simulink model "LogicalArch"  (R2025a)
settings: Solver=FixedStepDiscrete  StartTime=0.0  StopTime=10.0  RelTol=1e-3
undefined symbols (not defined in the file): D1, P
settings Model: DataDictionary=MotionController.sldd  Creator=mfussi  LastModifiedBy=mfussi
settings OptimizationCC: DefaultParameterBehavior=Inlined  EnhancedBackFolding=on  PassReuseOutputArgsAs=Individual arguments  ZeroExternalMemoryAtStartup=off  ZeroInternalMemoryAtStartup=off  OptimizeBlockOrder=speed  DifferentSizesBufferReuse=on  OptimizationCustomize=off  EfficientTunableParamExpr=on
settings DebuggingCC: ParameterTunabilityLossMsg=error
settings SFSimCC: MATLABDynamicMemAlloc=off
settings RTWCC: SystemTargetFile=ert.tlc  TemplateMakefile=ert_default_tmf  Description=Embedded Coder
settings CodeAppCC: ForceParamTrailComments=on  IgnoreCustomStorageClasses=off  OperatorAnnotations=on  SimulinkDataObjDesc=on  SFDataObjDesc=on  InsertBlockDesc=on
settings ERTTargetCC: ExtModeTransport=0.0  ExtModeStaticAlloc=off  ExtModeMexFile=ext_comm  ExtModeIntrfLevel=Level1  ERTCustomFileTemplate=example_file_process.tlc  TargetLangStandard=C99 (ISO)  GenerateSampleERTMain=on

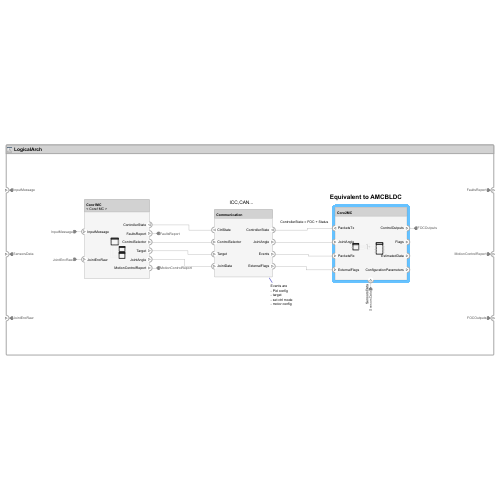
[thumbnail: Simulink's stored preview of the top-level diagram]
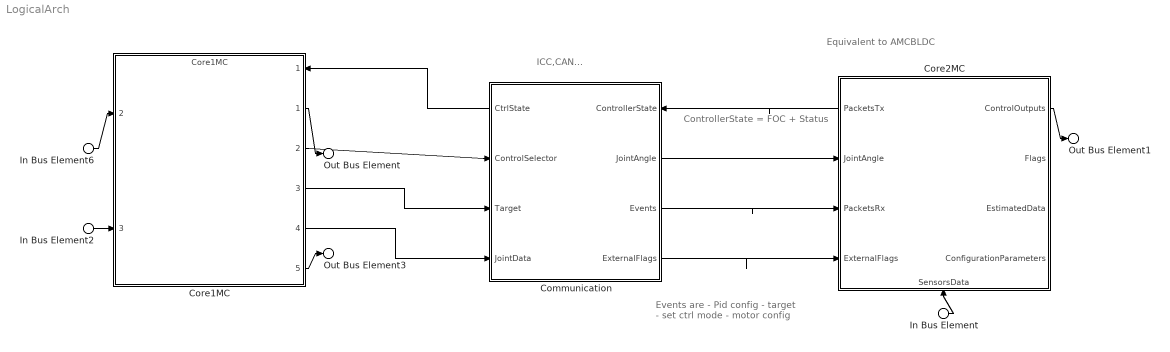
== system LogicalArch ==
  note: ControllerState = FOC + Status
  note: Events are
      | - Pid config
      | - target
      | - set ctrl mode
      | - motor config
  note: ICC,CAN...
  note: Equivalent to AMCBLDC
  In Bus Element6 : Inport  PortName=InputMessage
  In Bus Element : Inport  Port=2  PortName=SensorsData
  In Bus Element2 : Inport  Port=3  PortName=JointEncRaw
  Communication : Subsystem
      settings: PortSchema="{\"entries\":[{\"content\":{\"headerSize\":26,\"margin\":15,\"minimumSpacing\":25,\"sides\":[{\"content\":{\"connectorIds\":[\"Out1\",\"In2\",\"In3\",\"In4\"]},\"type\":\"ConnectorPlacement.EquallySpacedRectSide\",\"uuid\":\"fe08bce5-e822-4f40-96c8-d2e734a990df\"},{\"content\":{\"connectorIds\":[\"In1\",\"Out2\",\"Out4\",\"Out3\"],\"side\":\"RIGHT\"},\"type\":\"ConnectorPlacement.EquallySpacedRectSide\",\"uuid\":\"919d1c7d-1061-4f77-a351-e4b0010947a9\"},{\"content\":{\"side\":\"TOP\"},\"type\":\"ConnectorPlacement.EquallySpacedRectSide\",\"uuid\":\"ced767b1-6519-463a-89bd-856cb58a8166\"}]},\"type\":\"ConnectorPlacement.EquallySpacedConnector\",\"uuid\":\"cdf15350-aaf1-41b4-b116-0e65771ee3f3\"}],\"packageUris\":[\"http://schema.mathworks.com/mf0/Connector/R2020b\"],\"version\":\"1.0\"}"
  Core1MC : ModelReference  ModelNameDialog=Core1MC.slx  SimulationMode=Normal  ScheduleRates=on  ModelReferenceVersion=1.2
      settings: PortSchema="{\"entries\":[{\"content\":{\"headerSize\":38,\"margin\":15,\"minimumSpacing\":25,\"sides\":[{\"content\":{\"connectorIds\":[\"In2\",\"In3\"]},\"type\":\"ConnectorPlacement.EquallySpacedRectSide\",\"uuid\":\"f116faee-1f2a-4df9-9539-2b4210afeefe\"},{\"content\":{\"connectorIds\":[\"In1\",\"Out1\",\"Out2\",\"Out3\",\"Out4\",\"Out5\"],\"side\":\"RIGHT\"},\"type\":\"ConnectorPlacement.EquallySpacedRectSide\",\"uuid\":\"15bee73e-70ab-48d7-8ec7-8f9a927bc16b\"},{\"content\":{\"side\":\"TOP\"},\"type\":\"ConnectorPlacement.EquallySpacedRectSide\",\"uuid\":\"028c131f-52af-49f4-b789-e2e615b5b11c\"}]},\"type\":\"ConnectorPlacement.EquallySpacedConnector\",\"uuid\":\"2ab3b17c-88dc-4a6c-bd49-4ef3d2b344d3\"}],\"packageUris\":[\"http://schema.mathworks.com/mf0/Connector/R2020b\"],\"version\":\"1.0\"}"
  Core2MC : Subsystem
      settings: PortSchema="{\"entries\":[{\"content\":{\"headerSize\":26,\"margin\":15,\"minimumSpacing\":25,\"sides\":[{\"content\":{\"connectorIds\":[\"Out1\",\"In1\",\"In3\",\"In2\"]},\"type\":\"ConnectorPlacement.EquallySpacedRectSide\",\"uuid\":\"8a080317-9bcc-45dd-ad9c-7d7a1d267dc1\"},{\"content\":{\"connectorIds\":[\"Out2\",\"Out3\",\"Out4\",\"Out5\"],\"side\":\"RIGHT\"},\"type\":\"ConnectorPlacement.EquallySpacedRectSide\",\"uuid\":\"40b95da5-0e38-4058-8ebd-913319e6fe12\"},{\"content\":{\"side\":\"TOP\"},\"type\":\"ConnectorPlacement.EquallySpacedRectSide\",\"uuid\":\"880187c3-7d3f-4130-85c8-9403ff1f590f\"},{\"content\":{\"connectorIds\":[\"In4\"],\"side\":\"BOTTOM\"},\"type\":\"ConnectorPlacement.EquallySpacedRectSide\",\"uuid\":\"cb8d9f13-ba0e-48de-be5c-602b33a49657\"}]},\"type\":\"ConnectorPlacement.EquallySpacedConnector\",\"uuid\":\"156347fc-2d8f-4aa4-81e2-6bd9fedc9a5a\"}],\"packageUris\":[\"http://schema.mathworks.com/mf0/Connector/R2020b\"],\"version\":\"1.0\"}"
  Out Bus Element : Outport  PortName=FaultsReport
  Out Bus Element3 : Outport  Port=2  PortName=MotionControlReport
  Out Bus Element1 : Outport  Port=3  PortName=FOCOutputs
  wires:
  Communication/2(JointAngle) -> Core2MC/1(JointAngle)
  Communication/4(Events) -> Core2MC/3(PacketsRx)
  Core2MC/1(PacketsTx) -> Communication/1(ControllerState)
  Core1MC/2 -> Communication/2(ControlSelector)
  Core1MC/3 -> Communication/3(Target)
  Core1MC/4 -> Communication/4(JointData)
  Communication/1(CtrlState) -> Core1MC/1
  In Bus Element6/1 -> Core1MC/2
  In Bus Element2/1 -> Core1MC/3
  In Bus Element/1 -> Core2MC/4(SensorsData)
  Communication/3(ExternalFlags) -> Core2MC/2(ExternalFlags)
  Core2MC/2(ControlOutputs) -> Out Bus Element1/1
  Core1MC/1 -> Out Bus Element/1
  Core1MC/5 -> Out Bus Element3/1

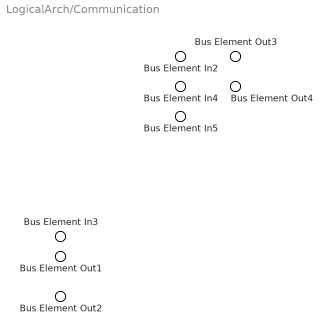
== system LogicalArch/Communication ==
  Bus Element In5 : Inport  PortName=ControllerState
  Bus Element In2 : Inport  Port=2  PortName=ControlSelector
  Bus Element In4 : Inport  Port=3  PortName=Target
  Bus Element In3 : Inport  Port=4  PortName=JointData
  Bus Element Out3 : Outport  PortName=CtrlState
  Bus Element Out1 : Outport  Port=2  PortName=JointAngle
  Bus Element Out4 : Outport  Port=3  PortName=ExternalFlags
  Bus Element Out2 : Outport  Port=4  PortName=Events

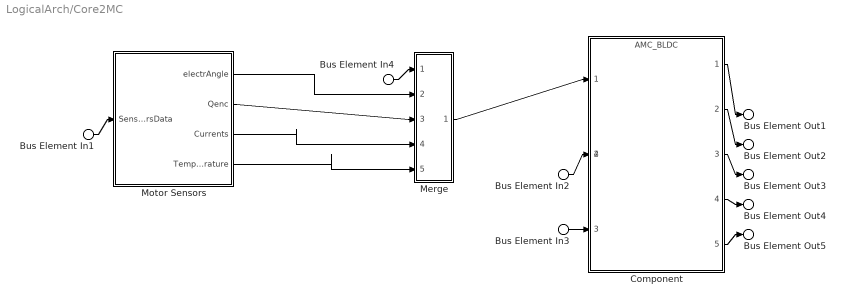
== system LogicalArch/Core2MC ==
  Bus Element In4 : Inport  PortName=JointAngle
  Bus Element In2 : Inport  Port=2  PortName=ExternalFlags
  Bus Element In3 : Inport  Port=3  PortName=PacketsRx
  Bus Element In1 : Inport  Port=4  PortName=SensorsData
  Component : ModelReference  ModelNameDialog=AMC_BLDC.slx  SimulationMode=Normal  ScheduleRates=on  ModelEventPortInfo=P:D1[-2][0][0]  ModelReferenceVersion=10.21
      settings: PortSchema="{\"entries\":[{\"content\":{\"headerSize\":38,\"margin\":15,\"minimumSpacing\":25,\"sides\":[{\"content\":{\"connectorIds\":[\"In1\",\"In2\",\"In3\"]},\"type\":\"ConnectorPlacement.EquallySpacedRectSide\",\"uuid\":\"f116faee-1f2a-4df9-9539-2b4210afeefe\"},{\"content\":{\"connectorIds\":[\"Out1\",\"Out2\",\"Out3\",\"Out4\",\"Out5\"],\"side\":\"RIGHT\"},\"type\":\"ConnectorPlacement.EquallySpacedRectSide\",\"uuid\":\"15bee73e-70ab-48d7-8ec7-8f9a927bc16b\"},{\"content\":{\"side\":\"TOP\"},\"type\":\"ConnectorPlacement.EquallySpacedRectSide\",\"uuid\":\"028c131f-52af-49f4-b789-e2e615b5b11c\"},{\"content\":{\"connectorIds\":[\"In4\"],\"side\":\"HIDDEN\"},\"type\":\"ConnectorPlacement.EquallySpacedRectSide\",\"uuid\":\"a9e6405e-7b1c-4ea5-9964-f820342ca78f\"}]},\"type\":\"ConnectorPlacement.EquallySpacedConnector\",\"uuid\":\"2ab3b17c-88dc-4a6c-bd49-4ef3d2b344d3\"}],\"packageUris\":[\"http://schema.mathworks.com/mf0/Connector/R2020b\"],\"version\":\"1.0\"}"
  Merge : Subsystem
      settings: PortSchema="{\"entries\":[{\"content\":{\"margin\":10,\"minimumSpacing\":15,\"sides\":[{\"content\":{\"connectorIds\":[\"In1\",\"In2\",\"In3\",\"In4\",\"In5\"]},\"type\":\"ConnectorPlacement.EquallySpacedRectSide\",\"uuid\":\"b721ea92-b23b-49c6-b256-e109cfde6d9a\"},{\"content\":{\"connectorIds\":[\"Out1\"],\"side\":\"RIGHT\"},\"type\":\"ConnectorPlacement.EquallySpacedRectSide\",\"uuid\":\"01ecff02-faf6-44fc-85cd-eb338f239b8b\"},{\"content\":{\"side\":\"TOP\"},\"type\":\"ConnectorPlacement.EquallySpacedRectSide\",\"uuid\":\"b7f583c7-535b-43ea-9e2b-1d6295f5e2cc\"}]},\"type\":\"ConnectorPlacement.EquallySpacedConnector\",\"uuid\":\"374a74ae-7551-4f3a-8e98-a33b88a70ffb\"}],\"packageUris\":[\"http://schema.mathworks.com/mf0/Connector/R2020b\"],\"version\":\"1.0\"}"
  Motor Sensors : Subsystem
      settings: PortSchema="{\"entries\":[{\"content\":{\"headerSize\":26,\"margin\":15,\"minimumSpacing\":25,\"sides\":[{\"content\":{\"connectorIds\":[\"In1\"]},\"type\":\"ConnectorPlacement.EquallySpacedRectSide\",\"uuid\":\"342e77a0-fe02-4293-9b8f-d7b4d9d1e449\"},{\"content\":{\"connectorIds\":[\"Out2\",\"Out3\",\"Out4\",\"Out1\"],\"side\":\"RIGHT\"},\"type\":\"ConnectorPlacement.EquallySpacedRectSide\",\"uuid\":\"44d1e335-dcc4-49cc-8b5e-810d6adc679c\"},{\"content\":{\"side\":\"TOP\"},\"type\":\"ConnectorPlacement.EquallySpacedRectSide\",\"uuid\":\"025af28e-bbdd-4ddf-9ce9-395878e2a87b\"},{\"content\":{\"side\":\"BOTTOM\"},\"type\":\"ConnectorPlacement.EquallySpacedRectSide\",\"uuid\":\"55873401-33e6-4ccb-9330-bdb43b58e7a9\"}]},\"type\":\"ConnectorPlacement.EquallySpacedConnector\",\"uuid\":\"48047874-33f0-4080-8e53-46ed85469308\"}],\"packageUris\":[\"http://schema.mathworks.com/mf0/Connector/R2020b\"],\"version\":\"1.0\"}"
  Bus Element Out5 : Outport  PortName=PacketsTx
  Bus Element Out1 : Outport  Port=2  PortName=ControlOutputs
  Bus Element Out3 : Outport  Port=3  PortName=Flags
  Bus Element Out4 : Outport  Port=4  PortName=EstimatedData
  Bus Element Out2 : Outport  Port=5  PortName=ConfigurationParameters
  wires:
  Bus Element In1/1 -> Motor Sensors/1(SensorsData)
  Motor Sensors/2(electrAngle) -> Merge/2(electrAngle)
  Motor Sensors/4(Currents) -> Merge/4(Currents)
  Motor Sensors/3(Qenc) -> Merge/3(Qenc)
  Motor Sensors/1(Temperature) -> Merge/5(Temperature)
  Merge/1(ProcessedSensors) -> Component/1
  Bus Element In2/1 -> Component/2
  Component/1 -> Bus Element Out1/1
  Component/2 -> Bus Element Out2/1
  Component/3 -> Bus Element Out3/1
  Component/4 -> Bus Element Out4/1
  Component/5 -> Bus Element Out5/1
  Bus Element In3/1 -> Component/3
  Bus Element In4/1 -> Merge/1(JointAngle)

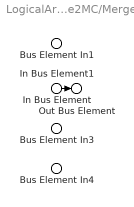
== system LogicalArch/Core2MC/Merge ==
  Bus Element In1 : Inport  PortName=JointAngle
  In Bus Element : Inport  Port=2  PortName=electrAngle
  In Bus Element1 : Inport  Port=3  PortName=Qenc
  Bus Element In3 : Inport  Port=4  PortName=Currents
  Bus Element In4 : Inport  Port=5  PortName=Temperature
  Out Bus Element : Outport  PortName=ProcessedSensors
  wires:
  In Bus Element/1 -> Out Bus Element/1

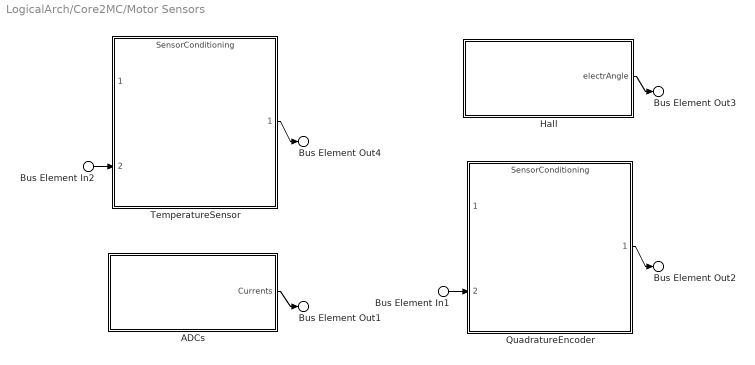
== system LogicalArch/Core2MC/Motor Sensors ==
  Bus Element In1 : Inport  PortName=SensorsData
  Bus Element In2 : Inport  PortName=SensorsData
  ADCs : Subsystem
      settings: PortSchema="{\"entries\":[{\"content\":{\"headerSize\":26,\"margin\":15,\"minimumSpacing\":25,\"sides\":[{\"content\":{},\"type\":\"ConnectorPlacement.EquallySpacedRectSide\",\"uuid\":\"15e2ce74-797f-4db5-be27-721c76b78586\"},{\"content\":{\"connectorIds\":[\"Out1\"],\"side\":\"RIGHT\"},\"type\":\"ConnectorPlacement.EquallySpacedRectSide\",\"uuid\":\"77d311f1-c2d5-4f29-9693-3cfe7ff3c66f\"},{\"content\":{\"side\":\"TOP\"},\"type\":\"ConnectorPlacement.EquallySpacedRectSide\",\"uuid\":\"0ad7fd31-5953-422f-9352-5b06c9bff885\"}]},\"type\":\"ConnectorPlacement.EquallySpacedConnector\",\"uuid\":\"9e5c4c0a-c38e-4cf1-bd50-bfe5cf75fba8\"}],\"packageUris\":[\"http://schema.mathworks.com/mf0/Connector/R2020b\"],\"version\":\"1.0\"}"
  Hall : Subsystem
      settings: PortSchema="{\"entries\":[{\"content\":{\"headerSize\":26,\"margin\":15,\"minimumSpacing\":25,\"sides\":[{\"content\":{},\"type\":\"ConnectorPlacement.EquallySpacedRectSide\",\"uuid\":\"fe08bce5-e822-4f40-96c8-d2e734a990df\"},{\"content\":{\"connectorIds\":[\"Out1\"],\"side\":\"RIGHT\"},\"type\":\"ConnectorPlacement.EquallySpacedRectSide\",\"uuid\":\"919d1c7d-1061-4f77-a351-e4b0010947a9\"},{\"content\":{\"side\":\"TOP\"},\"type\":\"ConnectorPlacement.EquallySpacedRectSide\",\"uuid\":\"ced767b1-6519-463a-89bd-856cb58a8166\"}]},\"type\":\"ConnectorPlacement.EquallySpacedConnector\",\"uuid\":\"cdf15350-aaf1-41b4-b116-0e65771ee3f3\"}],\"packageUris\":[\"http://schema.mathworks.com/mf0/Connector/R2020b\"],\"version\":\"1.0\"}"
  QuadratureEncoder : ModelReference  ModelNameDialog=SensorConditioning.slx  SimulationMode=Normal  ScheduleRates=on  ModelReferenceVersion=1.2
      settings: PortSchema="{\"entries\":[{\"content\":{\"headerSize\":38,\"margin\":15,\"minimumSpacing\":25,\"sides\":[{\"content\":{\"connectorIds\":[\"In1\",\"In2\"]},\"type\":\"ConnectorPlacement.EquallySpacedRectSide\",\"uuid\":\"6d6857fa-f5c9-43b4-a306-0920391a2fd0\"},{\"content\":{\"connectorIds\":[\"Out1\"],\"side\":\"RIGHT\"},\"type\":\"ConnectorPlacement.EquallySpacedRectSide\",\"uuid\":\"4567897e-6982-4f2c-af43-5ed4bc8792a2\"},{\"content\":{\"side\":\"TOP\"},\"type\":\"ConnectorPlacement.EquallySpacedRectSide\",\"uuid\":\"b9101744-fe35-433d-bb4c-e7449aefab81\"}]},\"type\":\"ConnectorPlacement.EquallySpacedConnector\",\"uuid\":\"96c92cf5-557b-4ff0-b6b4-f2ae6063b6b3\"}],\"packageUris\":[\"http://schema.mathworks.com/mf0/Connector/R2020b\"],\"version\":\"1.0\"}"
  TemperatureSensor : ModelReference  ModelNameDialog=SensorConditioning.slx  SimulationMode=Normal  ScheduleRates=on  ModelReferenceVersion=1.2
      settings: PortSchema="{\"entries\":[{\"content\":{\"headerSize\":38,\"margin\":15,\"minimumSpacing\":25,\"sides\":[{\"content\":{\"connectorIds\":[\"In1\",\"In2\"]},\"type\":\"ConnectorPlacement.EquallySpacedRectSide\",\"uuid\":\"6d6857fa-f5c9-43b4-a306-0920391a2fd0\"},{\"content\":{\"connectorIds\":[\"Out1\"],\"side\":\"RIGHT\"},\"type\":\"ConnectorPlacement.EquallySpacedRectSide\",\"uuid\":\"4567897e-6982-4f2c-af43-5ed4bc8792a2\"},{\"content\":{\"side\":\"TOP\"},\"type\":\"ConnectorPlacement.EquallySpacedRectSide\",\"uuid\":\"b9101744-fe35-433d-bb4c-e7449aefab81\"}]},\"type\":\"ConnectorPlacement.EquallySpacedConnector\",\"uuid\":\"96c92cf5-557b-4ff0-b6b4-f2ae6063b6b3\"}],\"packageUris\":[\"http://schema.mathworks.com/mf0/Connector/R2020b\"],\"version\":\"1.0\"}"
  Bus Element Out4 : Outport  PortName=Temperature
  Bus Element Out3 : Outport  Port=2  PortName=electrAngle
  Bus Element Out2 : Outport  Port=3  PortName=Qenc
  Bus Element Out1 : Outport  Port=4  PortName=Currents
  wires:
  ADCs/1(Currents) -> Bus Element Out1/1
  Hall/1(electrAngle) -> Bus Element Out3/1
  TemperatureSensor/1 -> Bus Element Out4/1
  QuadratureEncoder/1 -> Bus Element Out2/1
  Bus Element In1/1 -> QuadratureEncoder/2
  Bus Element In2/1 -> TemperatureSensor/2

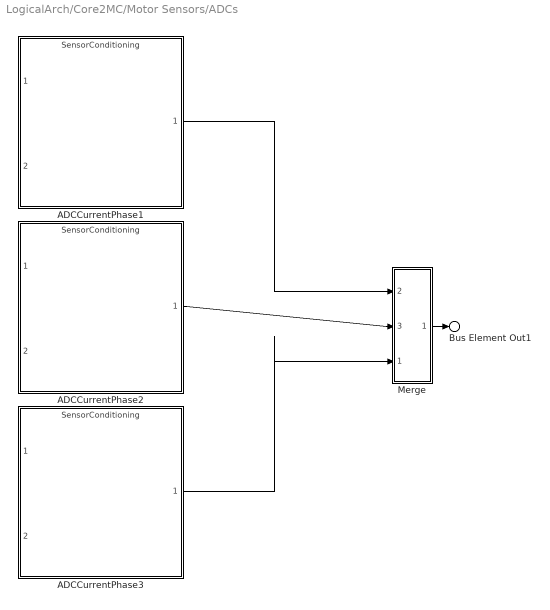
== system LogicalArch/Core2MC/Motor Sensors/ADCs ==
  ADCCurrentPhase1 : ModelReference  ModelNameDialog=SensorConditioning.slx  SimulationMode=Normal  ScheduleRates=on  ModelReferenceVersion=1.2
      settings: PortSchema="{\"entries\":[{\"content\":{\"headerSize\":38,\"margin\":15,\"minimumSpacing\":25,\"sides\":[{\"content\":{\"connectorIds\":[\"In1\",\"In2\"]},\"type\":\"ConnectorPlacement.EquallySpacedRectSide\",\"uuid\":\"6d6857fa-f5c9-43b4-a306-0920391a2fd0\"},{\"content\":{\"connectorIds\":[\"Out1\"],\"side\":\"RIGHT\"},\"type\":\"ConnectorPlacement.EquallySpacedRectSide\",\"uuid\":\"4567897e-6982-4f2c-af43-5ed4bc8792a2\"},{\"content\":{\"side\":\"TOP\"},\"type\":\"ConnectorPlacement.EquallySpacedRectSide\",\"uuid\":\"b9101744-fe35-433d-bb4c-e7449aefab81\"}]},\"type\":\"ConnectorPlacement.EquallySpacedConnector\",\"uuid\":\"96c92cf5-557b-4ff0-b6b4-f2ae6063b6b3\"}],\"packageUris\":[\"http://schema.mathworks.com/mf0/Connector/R2020b\"],\"version\":\"1.0\"}"
  ADCCurrentPhase2 : ModelReference  ModelNameDialog=SensorConditioning.slx  SimulationMode=Normal  ScheduleRates=on  ModelReferenceVersion=1.2
      settings: PortSchema="{\"entries\":[{\"content\":{\"headerSize\":38,\"margin\":15,\"minimumSpacing\":25,\"sides\":[{\"content\":{\"connectorIds\":[\"In1\",\"In2\"]},\"type\":\"ConnectorPlacement.EquallySpacedRectSide\",\"uuid\":\"6d6857fa-f5c9-43b4-a306-0920391a2fd0\"},{\"content\":{\"connectorIds\":[\"Out1\"],\"side\":\"RIGHT\"},\"type\":\"ConnectorPlacement.EquallySpacedRectSide\",\"uuid\":\"4567897e-6982-4f2c-af43-5ed4bc8792a2\"},{\"content\":{\"side\":\"TOP\"},\"type\":\"ConnectorPlacement.EquallySpacedRectSide\",\"uuid\":\"b9101744-fe35-433d-bb4c-e7449aefab81\"}]},\"type\":\"ConnectorPlacement.EquallySpacedConnector\",\"uuid\":\"96c92cf5-557b-4ff0-b6b4-f2ae6063b6b3\"}],\"packageUris\":[\"http://schema.mathworks.com/mf0/Connector/R2020b\"],\"version\":\"1.0\"}"
  ADCCurrentPhase3 : ModelReference  ModelNameDialog=SensorConditioning.slx  SimulationMode=Normal  ScheduleRates=on  ModelReferenceVersion=1.2
      settings: PortSchema="{\"entries\":[{\"content\":{\"headerSize\":38,\"margin\":15,\"minimumSpacing\":25,\"sides\":[{\"content\":{\"connectorIds\":[\"In1\",\"In2\"]},\"type\":\"ConnectorPlacement.EquallySpacedRectSide\",\"uuid\":\"6d6857fa-f5c9-43b4-a306-0920391a2fd0\"},{\"content\":{\"connectorIds\":[\"Out1\"],\"side\":\"RIGHT\"},\"type\":\"ConnectorPlacement.EquallySpacedRectSide\",\"uuid\":\"4567897e-6982-4f2c-af43-5ed4bc8792a2\"},{\"content\":{\"side\":\"TOP\"},\"type\":\"ConnectorPlacement.EquallySpacedRectSide\",\"uuid\":\"b9101744-fe35-433d-bb4c-e7449aefab81\"}]},\"type\":\"ConnectorPlacement.EquallySpacedConnector\",\"uuid\":\"96c92cf5-557b-4ff0-b6b4-f2ae6063b6b3\"}],\"packageUris\":[\"http://schema.mathworks.com/mf0/Connector/R2020b\"],\"version\":\"1.0\"}"
  Merge : Subsystem
      settings: PortSchema="{\"entries\":[{\"content\":{\"margin\":10,\"minimumSpacing\":15,\"sides\":[{\"content\":{\"connectorIds\":[\"In2\",\"In3\",\"In1\"]},\"type\":\"ConnectorPlacement.EquallySpacedRectSide\",\"uuid\":\"7f12f04c-5461-4836-a734-adc2bf884dca\"},{\"content\":{\"connectorIds\":[\"Out1\"],\"side\":\"RIGHT\"},\"type\":\"ConnectorPlacement.EquallySpacedRectSide\",\"uuid\":\"3e6e724d-a2e9-44fd-aa47-81a7ca7b1e30\"},{\"content\":{\"side\":\"TOP\"},\"type\":\"ConnectorPlacement.EquallySpacedRectSide\",\"uuid\":\"a6eebf31-70f0-4364-98fd-7bcbddea794c\"},{\"content\":{\"side\":\"BOTTOM\"},\"type\":\"ConnectorPlacement.EquallySpacedRectSide\",\"uuid\":\"70e5c21f-7bf5-4633-9f55-33f7ef1ae04e\"}]},\"type\":\"ConnectorPlacement.EquallySpacedConnector\",\"uuid\":\"958be322-7dc9-477a-a570-cb6c9a7ff655\"}],\"packageUris\":[\"http://schema.mathworks.com/mf0/Connector/R2020b\"],\"version\":\"1.0\"}"
  Bus Element Out1 : Outport  PortName=Currents
  wires:
  Merge/1(Currents) -> Bus Element Out1/1
  ADCCurrentPhase1/1 -> Merge/2("CurrentPhase1 ")
  ADCCurrentPhase2/1 -> Merge/3(CurrentPhase2)
  ADCCurrentPhase3/1 -> Merge/1(CurrentPhase3)

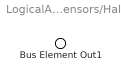
== system LogicalArch/Core2MC/Motor Sensors/Hall ==
  Bus Element Out1 : Outport  PortName=electrAngle

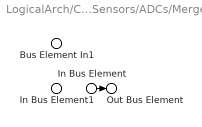
== system LogicalArch/Core2MC/Motor Sensors/ADCs/Merge ==
  Bus Element In1 : Inport  PortName=CurrentPhase3
  In Bus Element : Inport  Port=2  PortName=CurrentPhase1
  In Bus Element1 : Inport  Port=3  PortName=CurrentPhase2
  Out Bus Element : Outport  PortName=Currents
  wires:
  In Bus Element/1 -> Out Bus Element/1
